simulink model "teseo"  (R2018a)
settings: Solver=FixedStepDiscrete  StartTime=0.0  StopTime=inf  FixedStep=0.1  RelTol=1e-3
model workspace (MAT data in the model file):
  SL_ROS_VariableLengthArrays_MaxSizes.CommonInfo.ArrayTruncateAction = 'EmitWarning'
  SL_ROS_VariableLengthArrays_MaxSizes.MsgTypeMap = containers.Map
  SL_ROS_VariableLengthArrays_MaxSizes.MsgTypeMap.serialization.keys = {'sensor_msgs/LaserScan'}
  SL_ROS_VariableLengthArrays_MaxSizes.MsgTypeMap.serialization.values{1}(1).PropertyName = 'Intensities'
  SL_ROS_VariableLengthArrays_MaxSizes.MsgTypeMap.serialization.values{1}(1).DataType = 'single'
  SL_ROS_VariableLengthArrays_MaxSizes.MsgTypeMap.serialization.values{1}(1).MaxLength = 360
  SL_ROS_VariableLengthArrays_MaxSizes.MsgTypeMap.serialization.values{1}(2).PropertyName = 'Ranges'
  SL_ROS_VariableLengthArrays_MaxSizes.MsgTypeMap.serialization.values{1}(2).DataType = 'single'
  SL_ROS_VariableLengthArrays_MaxSizes.MsgTypeMap.serialization.values{1}(2).MaxLength = 360
  SL_ROS_VariableLengthArrays_MaxSizes.MsgTypeMap.serialization.uniformity = 0
  SL_ROS_VariableLengthArrays_MaxSizes.MsgTypeMap.serialization.keyType = 'char'
  SL_ROS_VariableLengthArrays_MaxSizes.MsgTypeMap.serialization.valueType = 'any'
undefined symbols (not defined in the file or in its folder): Angular, anti_gain, Linear, max_vel
libraries: simulink x9, robotlib x5
settings Model: EnablePacing=on  PacingRate=10  Creator=Daniele  LastModifiedBy=gabriele
settings RTWCC: Description=Generic Real-Time Target  RTWCompilerOptimization=on
settings CodeAppCC: MaxIdLength=95  StateflowObjectComments=on

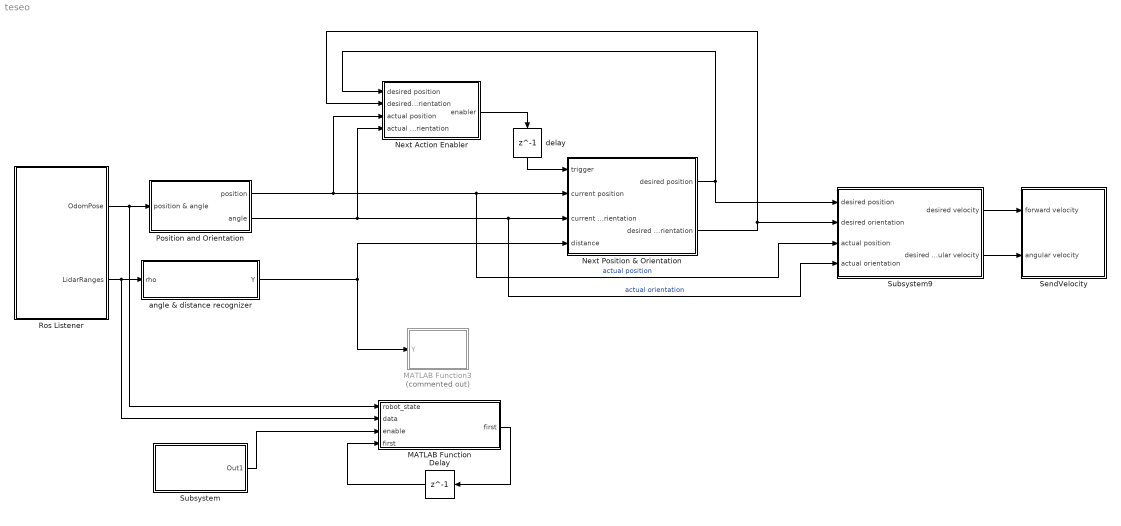
== system teseo ==
  Delay : Delay  DelayLength=1  InitialCondition=true
  MATLAB Function : MATLAB Function  TreatAsAtomicUnit=on
  MATLAB Function3 : MATLAB Function  Commented=on  TreatAsAtomicUnit=on
  Next Action Enabler : Subsystem
  Next Position & Orientation : Subsystem  mask{separation=0.5, offset=0, angle=2/9}
      mask prompts: separation "Distance between walls"; offset "Offset with respect to axes"; angle "Width of lateral angle: pi *"
  Position and Orientation : Subsystem
      mask Display:
      | disp('Pos/Angle\nSplitter')
      | port_label('input', 1, '[x y \theta]', 'interpreter', 'tex');
      | port_label('output', 1, '[x y]', 'interpreter', 'tex');
      | port_label('output', 2, '\theta', 'interpreter', 'tex');
  Ros Listener : Subsystem
  SendVelocity : Subsystem
  Subsystem : Subsystem
      mask Display: fprintf('Iteration Counter')
  Subsystem9 : Subsystem
  angle & distance recognizer : MATLAB Function  TreatAsAtomicUnit=on
  delay : Delay  DelayLength=1  InitialCondition=1
  wires:
  Ros Listener/1(OdomPose) -> MATLAB Function/1(robot_state), Position and Orientation/1(position & angle)
  Position and Orientation/1(position) -> Subsystem9/3(actual position), Next Position & Orientation/2(current position), Next Action Enabler/3(actual position)  "actual position"
  Position and Orientation/2(angle) -> Subsystem9/4(actual orientation), Next Position & Orientation/3(current orientation), Next Action Enabler/4(actual orientation)  "actual orientation"
  Ros Listener/2(LidarRanges) -> MATLAB Function/2(data), angle & distance recognizer/1(rho)
  angle & distance recognizer/1(Y) -> MATLAB Function3/1(Y), Next Position & Orientation/4(distance)
  delay/1 -> Next Position & Orientation/1(trigger)
  Next Action Enabler/1(enabler) -> delay/1
  Next Position & Orientation/1(desired position) -> Subsystem9/1(desired position), Next Action Enabler/1(desired position)
  Next Position & Orientation/2(desired orientation) -> Next Action Enabler/2(desired orientation), Subsystem9/2(desired orientation)
  Subsystem9/2(desired angular velocity) -> SendVelocity/2(angular velocity)
  Subsystem9/1(desired velocity) -> SendVelocity/1(forward velocity)
  Delay/1 -> MATLAB Function/4("first ")
  MATLAB Function/1(first) -> Delay/1
  Subsystem/1(Out1) -> MATLAB Function/3(enable)

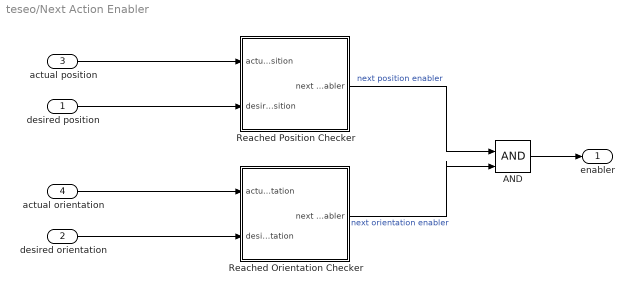
== system teseo/Next Action Enabler ==
  desired position : Inport
  desired orientation : Inport  Port=2
  actual position : Inport  Port=3
  actual orientation : Inport  Port=4
  AND : Logic  IconShape=distinctive  AllPortsSameDT=off  OutDataTypeStr=boolean
  Reached Orientation Checker : Subsystem  mask{stop_threshold=0.05, time_threshold=150}
      mask prompts: stop_threshold "Stop Threshold"; time_threshold "Time Threshold"
  Reached Position Checker : Subsystem  mask{stop_threshold=0.05, time_threshold=150}
      mask prompts: stop_threshold "Stop Treshold"; time_threshold "Time Treshold"
  enabler : Outport
  wires:
  actual orientation/1 -> Reached Orientation Checker/1(actual orientation)
  Reached Orientation Checker/1(next orientation enabler) -> AND/2  "next orientation enabler"
  Reached Position Checker/1(next position enabler) -> AND/1  "next position enabler"
  desired position/1 -> Reached Position Checker/2(desired position)
  desired orientation/1 -> Reached Orientation Checker/2(desired orientation)
  AND/1 -> enabler/1
  actual position/1 -> Reached Position Checker/1(actual position)

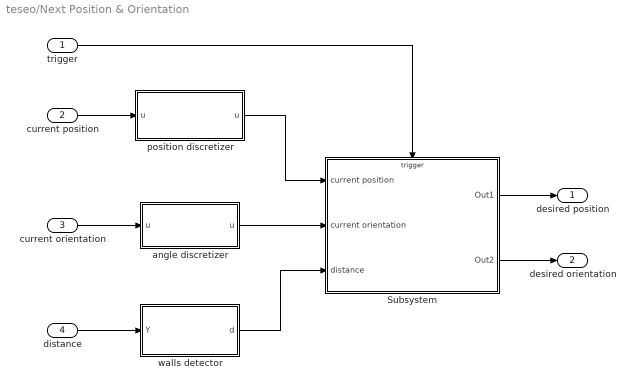
== system teseo/Next Position & Orientation ==
  trigger : Inport
  current position : Inport  Port=2
  current orientation : Inport  Port=3
  distance : Inport  Port=4
  Subsystem : Subsystem
  angle discretizer : MATLAB Function  TreatAsAtomicUnit=on
  position discretizer : MATLAB Function  TreatAsAtomicUnit=on  mask{width=separation, offset=offset}
      mask prompts: width "Distance between walls"; offset "Offset with respect to axes"
  walls detector : MATLAB Function  TreatAsAtomicUnit=on  mask{w=angle}
      mask prompts: w "Width of lateral angle"
  desired position : Outport
  desired orientation : Outport  Port=2
  wires:
  distance/1 -> walls detector/1(Y)
  current orientation/1 -> angle discretizer/1("u ")
  current position/1 -> position discretizer/1("u ")
  position discretizer/1(u) -> Subsystem/1(current position)
  angle discretizer/1(u) -> Subsystem/2(current orientation)
  walls detector/1(d) -> Subsystem/3(distance)
  Subsystem/1(Out1) -> desired position/1
  Subsystem/2(Out2) -> desired orientation/1
  trigger/1 -> Subsystem/Trigger

== system teseo/Position and Orientation ==
  position & angle : Inport
  Demux : Demux  Outputs=3
  Mux : Mux  Inputs=2
  position : Outport
  angle : Outport  Port=2
  wires:
  Demux/2 -> Mux/2
  position & angle/1 -> Demux/1
  Demux/1 -> Mux/1
  Mux/1 -> position/1
  Demux/3 -> angle/1

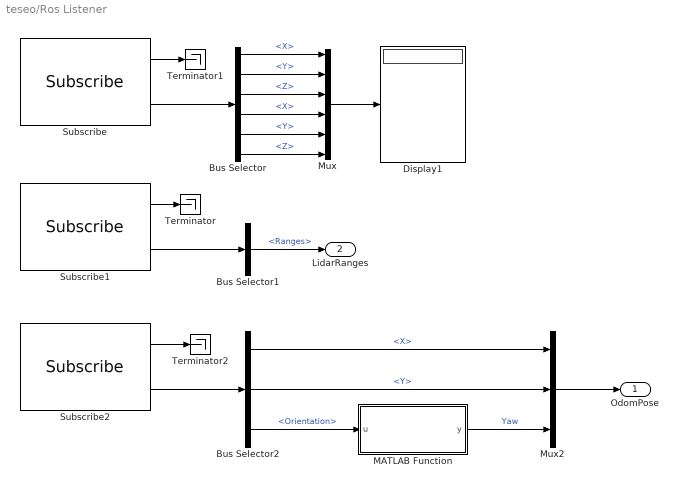
== system teseo/Ros Listener ==
  Bus Selector : BusSelector  OutputSignals=Linear.X,Linear.Y,Linear.Z,Angular.X,Angular.Y,Angular.Z
  Bus Selector1 : BusSelector  OutputSignals=Ranges
  Bus Selector2 : BusSelector  OutputSignals=Pose.Pose.Position.X,Pose.Pose.Position.Y,Pose.Pose.Orientation
  Display1 : Display
  MATLAB Function : MATLAB Function  TreatAsAtomicUnit=on
  Mux : Mux  Inputs=6
  Mux2 : Mux  Inputs=3
  Subscribe : robotlib/Subscribe  SourceLibraryInfo=This block requires Robotics System Toolbox  topicSource=Select from ROS network  topic=/mobile_base/commands/velocity  messageType=geometry_msgs/Twist  sampleTime=-1  messageQueueLength=1
      settings: SourceProductBaseCode=RO
  Subscribe1 : robotlib/Subscribe  SourceLibraryInfo=This block requires Robotics System Toolbox  topicSource=Select from ROS network  topic=/scan  messageType=sensor_msgs/LaserScan  sampleTime=-1  messageQueueLength=1
      settings: SourceProductBaseCode=RO
  Subscribe2 : robotlib/Subscribe  SourceLibraryInfo=This block requires Robotics System Toolbox  topicSource=Select from ROS network  topic=/odom  messageType=nav_msgs/Odometry  sampleTime=-1  messageQueueLength=1
      settings: SourceProductBaseCode=RO
  Terminator : Terminator
  Terminator1 : Terminator
  Terminator2 : Terminator
  OdomPose : Outport
  LidarRanges : Outport  Port=2
  wires:
  Bus Selector1/1 -> LidarRanges/1  "<Ranges>"
  Subscribe1/2 -> Bus Selector1/1
  Subscribe2/2 -> Bus Selector2/1
  Bus Selector2/1 -> Mux2/1  "<X>"
  Bus Selector2/2 -> Mux2/2  "<Y>"
  Mux2/1 -> OdomPose/1
  Bus Selector/5 -> Mux/5  "<Y>"
  Bus Selector/2 -> Mux/2  "<Y>"
  Bus Selector/1 -> Mux/1  "<X>"
  Bus Selector/6 -> Mux/6  "<Z>"
  Bus Selector/4 -> Mux/4  "<X>"
  Bus Selector/3 -> Mux/3  "<Z>"
  Mux/1 -> Display1/1
  Subscribe/2 -> Bus Selector/1
  Bus Selector2/3 -> MATLAB Function/1(u)  "<Orientation>"
  MATLAB Function/1(y) -> Mux2/3  "Yaw"
  Subscribe1/1 -> Terminator/1
  Subscribe/1 -> Terminator1/1
  Subscribe2/1 -> Terminator2/1

== system teseo/SendVelocity ==
  forward velocity : Inport
  angular velocity : Inport  Port=2
  Blank Message1 : robotlib/Blank Message  SourceLibraryInfo=This block requires Robotics System Toolbox  messageType=geometry_msgs/Twist  SampleTime=-1
      settings: SourceProductBaseCode=RO
  Bus Assignment1 : BusAssignment  AssignedSignals=Linear.X,Angular.Z
  Publish1 : robotlib/Publish  SourceLibraryInfo=This block requires Robotics System Toolbox  topicSource=Select from ROS network  topic=/cmd_vel  messageType=geometry_msgs/Twist  messageQueueLength=5
      settings: SourceProductBaseCode=RO
  wires:
  Blank Message1/1 -> Bus Assignment1/1
  forward velocity/1 -> Bus Assignment1/2
  angular velocity/1 -> Bus Assignment1/3
  Bus Assignment1/1 -> Publish1/1

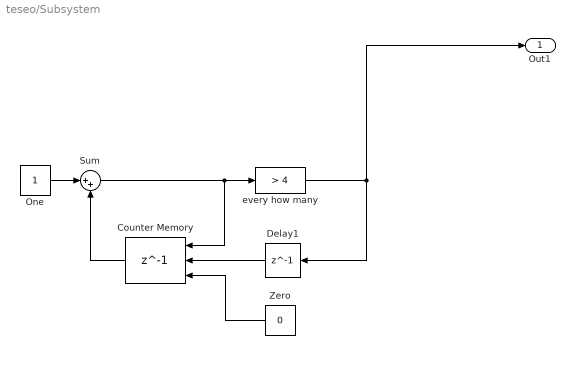
== system teseo/Subsystem ==
  Counter Memory : Delay  DelayLength=1  InitialConditionSource=Input port  ExternalReset=Rising
      settings: InputPortMap=u0,r5,p4
  Delay1 : Delay  DelayLength=1  InitialCondition=false
  One : Constant
  Sum : Sum  Inputs=|++
  Zero : Constant  Value=0
  every how many : simulink/Logic and Bit Operations/Compare To Constant  relop=>  const=4  OutDataTypeStr=boolean
  Out1 : Outport
  wires:
  Zero/1 -> Counter Memory/3
  Sum/1 -> every how many/1, Counter Memory/1
  Delay1/1 -> Counter Memory/2
  Counter Memory/1 -> Sum/2
  every how many/1 -> Out1/1, Delay1/1
  One/1 -> Sum/1

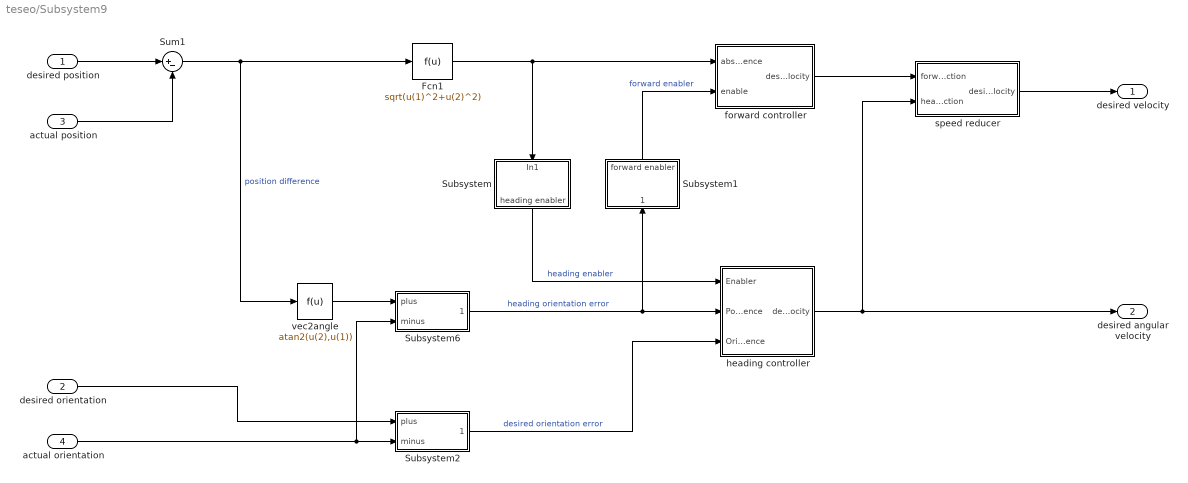
== system teseo/Subsystem9 ==
  desired position : Inport
  desired orientation : Inport  Port=2
  actual position : Inport  Port=3
  actual orientation : Inport  Port=4
  Fcn1 : Fcn  Expr=sqrt(u(1)^2+u(2)^2)
      mask Display: disp('norm')
  Subsystem : Subsystem  mask{heading_en_threshold=0.05}
      mask prompts: heading_en_threshold "Heading Enabler Threshold: |u| >"
      mask Display: fprintf("Heading\nEnabler")
  Subsystem1 : Subsystem  mask{forward_en_threshold=0.2}
      mask prompts: forward_en_threshold "Forward Motion Enabler Threshold: |u| <"
      mask Display: fprintf("Forward\nEnabler")
  Subsystem2 : Subsystem
      mask Display:
      | disp('anglediff');
      | port_label('input', 1, '+');
      | port_label('input', 2, '-');
  Subsystem6 : Subsystem
      mask Display:
      | disp('anglediff');
      | port_label('input', 1, '+');
      | port_label('input', 2, '-');
  Sum1 : Sum  Inputs=|+-
  forward controller : Subsystem  mask{gain=2, int_gain=0, der_gain=0.5}
      mask prompts: gain "Proportional Gain"; int_gain "Integral Gain"; der_gain "Derivative Gain"
      mask Display: disp('Forward Motion\nController')
  heading controller : Subsystem  mask{gain=2, int_gain=0, der_gain=1}
      mask prompts: gain "Proportional Gain"; int_gain "Integral Gain"; der_gain "Derivative Gain"
      mask Display: disp('Yaw Controller')
  speed reducer : Subsystem  mask{speed_red_threshold=0.5, low_speed=0.5, high_speed=0.75}
      mask prompts: speed_red_threshold "Speed Reducer Threshold: |heading action| >"; low_speed "Low Speed Multiplier"; high_speed "High Speed Multiplier"
      mask Display: fprintf("Speed Reducer")
  vec2angle : Fcn  Expr=atan2(u(2),u(1))
      mask Display: disp('angle')
  desired velocity : Outport
  desired angular velocity : Outport  Port=2
  wires:
  vec2angle/1 -> Subsystem6/1("plus ")
  heading controller/1(desired angular velocity) -> speed reducer/2(heading action), desired angular velocity/1
  actual orientation/1 -> Subsystem2/2(minus), Subsystem6/2(minus)
  desired orientation/1 -> Subsystem2/1("plus ")
  desired position/1 -> Sum1/1
  Sum1/1 -> vec2angle/1, Fcn1/1  "position difference"
  Subsystem2/1(difference) -> heading controller/3(Orientation Angular Difference)  "desired orientation error"
  actual position/1 -> Sum1/2
  Fcn1/1 -> Subsystem/1(In1), forward controller/1(absolute position difference)
  Subsystem6/1(difference) -> heading controller/2(Position Angular Difference), Subsystem1/1(heading orientation error)  "heading orientation error"
  forward controller/1(desired velocity) -> speed reducer/1(forward action)
  speed reducer/1(desired velocity) -> desired velocity/1
  Subsystem/1(heading enabler) -> heading controller/1(Enabler)  "heading enabler"
  Subsystem1/1(forward enabler) -> forward controller/2(enable)  "forward enabler"

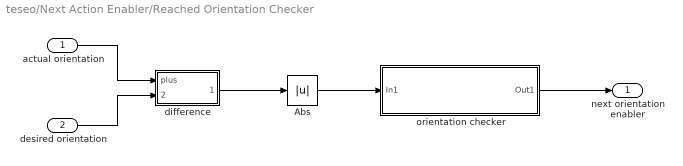
== system teseo/Next Action Enabler/Reached Orientation Checker ==
  actual orientation : Inport
  desired orientation : Inport  Port=2
  Abs : Abs
  difference : Subsystem
      mask Display: disp('anglediff')
  orientation checker : Subsystem  mask{stop_treshold=stop_threshold, time_threshold=time_threshold}
      mask prompts: stop_treshold "Stop Threshold"; time_threshold "Time Threshold"
      mask Display: fprintf("Reached Destination Checker");
  next orientation enabler : Outport
  wires:
  difference/1(difference) -> Abs/1
  Abs/1 -> orientation checker/1(In1)
  orientation checker/1(Out1) -> next orientation enabler/1
  actual orientation/1 -> difference/1("plus ")
  desired orientation/1 -> difference/2(minus)

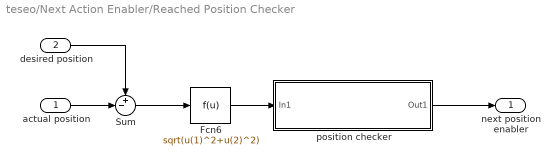
== system teseo/Next Action Enabler/Reached Position Checker ==
  actual position : Inport
  desired position : Inport  Port=2
  Fcn6 : Fcn  Expr=sqrt(u(1)^2+u(2)^2)
      mask Display: disp('norm')
  Sum : Sum  Inputs=+-|
  position checker : Subsystem  mask{stop_treshold=stop_threshold, time_threshold=time_threshold}
      mask prompts: stop_treshold "Stop Threshold"; time_threshold "Time Threshold"
      mask Display: fprintf("Reached Destination Checker");
  next position enabler : Outport
  wires:
  Fcn6/1 -> position checker/1(In1)
  Sum/1 -> Fcn6/1
  actual position/1 -> Sum/2
  desired position/1 -> Sum/1
  position checker/1(Out1) -> next position enabler/1

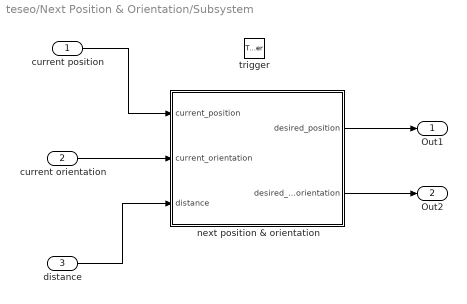
== system teseo/Next Position & Orientation/Subsystem ==
  current position : Inport
  current orientation : Inport  Port=2
  distance : Inport  Port=3
  trigger : TriggerPort  VariantControl=Variant  InitialTriggerSignalState=zero  PortDimensions=1
  next position & orientation : MATLAB Function  TreatAsAtomicUnit=on
  Out1 : Outport
  Out2 : Outport  Port=2
  wires:
  current orientation/1 -> next position & orientation/2(current_orientation)
  distance/1 -> next position & orientation/3(distance)
  next position & orientation/2(desired_orientation) -> Out2/1
  next position & orientation/1(desired_position) -> Out1/1
  current position/1 -> next position & orientation/1(current_position)

== system teseo/Subsystem9/Subsystem ==
  In1 : Inport
  Abs : Abs
  Compare To Constant : simulink/Logic and Bit Operations/Compare To Constant  relop=>  const=heading_en_threshold  OutDataTypeStr=boolean
  heading enabler : Outport
  wires:
  Compare To Constant/1 -> heading enabler/1
  In1/1 -> Abs/1
  Abs/1 -> Compare To Constant/1

== system teseo/Subsystem9/Subsystem1 ==
  heading orientation error : Inport
  Abs : Abs
  Compare To Constant : simulink/Logic and Bit Operations/Compare To Constant  relop=<  const=forward_en_threshold  OutDataTypeStr=boolean
  forward enabler : Outport
  wires:
  heading orientation error/1 -> Abs/1
  Compare To Constant/1 -> forward enabler/1
  Abs/1 -> Compare To Constant/1

== system teseo/Subsystem9/Subsystem2 ==
  "plus " : Inport
  minus : Inport  Port=2
  MATLAB Function : MATLAB Function  TreatAsAtomicUnit=on
  Mux : Mux  Inputs=2
  difference : Outport
  wires:
  MATLAB Function/1(y) -> difference/1
  Mux/1 -> MATLAB Function/1(u)
  "plus "/1 -> Mux/2
  minus/1 -> Mux/1

== system teseo/Subsystem9/Subsystem6 ==
  "plus " : Inport
  minus : Inport  Port=2
  MATLAB Function : MATLAB Function  TreatAsAtomicUnit=on
  Mux : Mux  Inputs=2
  difference : Outport
  wires:
  MATLAB Function/1(y) -> difference/1
  Mux/1 -> MATLAB Function/1(u)
  "plus "/1 -> Mux/2
  minus/1 -> Mux/1

== system teseo/Subsystem9/forward controller ==
  absolute position difference : Inport
  enable : Inport  Port=2
  PID Controller : simulink/Continuous/PID Controller  Controller=PID  TimeDomain=Discrete-time  SampleTime=-1  IntegratorMethod=Forward Euler  FilterMethod=Trapezoidal  Form=Parallel  UseFilter=on  ControllerParametersSource=internal  P=gain  I=int_gain  D=der_gain  N=100  InitialConditionSource=internal  InitialConditionForIntegrator=0  InitialConditionForFilter=0  ExternalReset=none  LimitOutput=off  UpperSaturationLimit=max_vel  LowerSaturationLimit=-max_vel  LinearizeAsGain=on  AntiWindupMode=back-calculation  Kb=anti_gain  TrackingMode=off  Kt=1  PParamMin=[]  PParamMax=[]  IParamMin=[]  IParamMax=[]  DParamMin=[]  DParamMax=[]  NParamMin=[]  NParamMax=[]  KbParamMin=[]  KbParamMax=[]  KtParamMin=[]  KtParamMax=[]  POutMin=[]  POutMax=[]  IOutMin=[]  IOutMax=[]  DOutMin=[]  DOutMax=[]  NOutMin=[]  NOutMax=[]  KbOutMin=[]  KbOutMax=[]  KtOutMin=[]  KtOutMax=[]  IntegratorOutMin=[]  IntegratorOutMax=[]  FilterOutMin=[]  FilterOutMax=[]  SumOutMin=[]  SumOutMax=[]  SumI1OutMin=[]  SumI1OutMax=[]  SumI2OutMin=[]  SumI2OutMax=[]  SumI3OutMin=[]  SumI3OutMax=[]  SumDOutMin=[]  SumDOutMax=[]  SaturationOutMin=[]  SaturationOutMax=[]  IntegratorContinuousStateAttributes=''  IntegratorStateMustResolveToSignalObject=off  IntegratorRTWStateStorageClass=Auto  FilterContinuousStateAttributes=''  FilterStateMustResolveToSignalObject=off  FilterRTWStateStorageClass=Auto  DifferentiatorICPrevScaledInput=0  DifferentiatorOutMin=[]  DifferentiatorOutMax=[]  FilterDiffOutCoefMin=[]  FilterDiffOutCoefMax=[]  SumDenOutMin=[]  SumDenOutMax=[]  SumNumOutMin=[]  SumNumOutMax=[]  ReciprocalOutMin=[]  ReciprocalOutMax=[]  DivideOutMin=[]  DivideOutMax=[]  TunerSelectOption=Frequency Response Based
  Switch2 : Switch
  zero : Constant  Value=0
  desired velocity : Outport
  wires:
  zero/1 -> Switch2/3
  Switch2/1 -> PID Controller/1
  enable/1 -> Switch2/2
  absolute position difference/1 -> Switch2/1
  PID Controller/1 -> desired velocity/1

== system teseo/Subsystem9/heading controller ==
  Enabler : Inport
  Position Angular Difference : Inport  Port=2
  Orientation Angular Difference : Inport  Port=3
  PID Controller : simulink/Continuous/PID Controller  Controller=PID  TimeDomain=Discrete-time  SampleTime=-1  IntegratorMethod=Trapezoidal  FilterMethod=Trapezoidal  Form=Parallel  UseFilter=on  ControllerParametersSource=internal  P=gain  I=int_gain  D=der_gain  N=100  InitialConditionSource=internal  InitialConditionForIntegrator=0  InitialConditionForFilter=0  ExternalReset=none  LimitOutput=off  UpperSaturationLimit=inf  LowerSaturationLimit=-inf  LinearizeAsGain=on  AntiWindupMode=none  Kb=1  TrackingMode=off  Kt=1  PParamMin=[]  PParamMax=[]  IParamMin=[]  IParamMax=[]  DParamMin=[]  DParamMax=[]  NParamMin=[]  NParamMax=[]  KbParamMin=[]  KbParamMax=[]  KtParamMin=[]  KtParamMax=[]  POutMin=[]  POutMax=[]  IOutMin=[]  IOutMax=[]  DOutMin=[]  DOutMax=[]  NOutMin=[]  NOutMax=[]  KbOutMin=[]  KbOutMax=[]  KtOutMin=[]  KtOutMax=[]  IntegratorOutMin=[]  IntegratorOutMax=[]  FilterOutMin=[]  FilterOutMax=[]  SumOutMin=[]  SumOutMax=[]  SumI1OutMin=[]  SumI1OutMax=[]  SumI2OutMin=[]  SumI2OutMax=[]  SumI3OutMin=[]  SumI3OutMax=[]  SumDOutMin=[]  SumDOutMax=[]  SaturationOutMin=[]  SaturationOutMax=[]  IntegratorContinuousStateAttributes=''  IntegratorStateMustResolveToSignalObject=off  IntegratorRTWStateStorageClass=Auto  FilterContinuousStateAttributes=''  FilterStateMustResolveToSignalObject=off  FilterRTWStateStorageClass=Auto  DifferentiatorICPrevScaledInput=0  DifferentiatorOutMin=[]  DifferentiatorOutMax=[]  FilterDiffOutCoefMin=[]  FilterDiffOutCoefMax=[]  SumDenOutMin=[]  SumDenOutMax=[]  SumNumOutMin=[]  SumNumOutMax=[]  ReciprocalOutMin=[]  ReciprocalOutMax=[]  DivideOutMin=[]  DivideOutMax=[]  TunerSelectOption=Frequency Response Based
  Switch : Switch
  desired angular velocity : Outport
  wires:
  Position Angular Difference/1 -> Switch/1
  PID Controller/1 -> desired angular velocity/1
  Switch/1 -> PID Controller/1
  Orientation Angular Difference/1 -> Switch/3
  Enabler/1 -> Switch/2

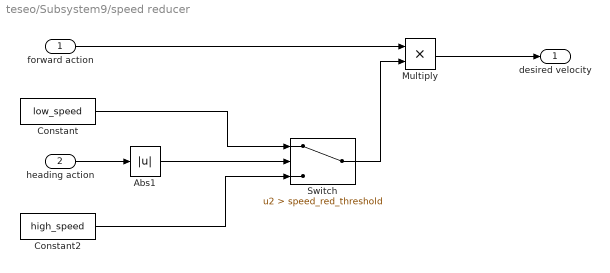
== system teseo/Subsystem9/speed reducer ==
  forward action : Inport
  heading action : Inport  Port=2
  Abs1 : Abs
  Constant : Constant  Value=low_speed
  Constant2 : Constant  Value=high_speed
  Multiply : Product
  Switch : Switch  Criteria=u2 > Threshold  Threshold=speed_red_threshold
  desired velocity : Outport
  wires:
  forward action/1 -> Multiply/1
  Switch/1 -> Multiply/2
  Constant2/1 -> Switch/3
  Multiply/1 -> desired velocity/1
  heading action/1 -> Abs1/1
  Abs1/1 -> Switch/2
  Constant/1 -> Switch/1

== system teseo/Next Action Enabler/Reached Orientation Checker/difference ==
  "plus " : Inport
  minus : Inport  Port=2
  MATLAB Function : MATLAB Function  TreatAsAtomicUnit=on
  Mux : Mux  Inputs=2
  difference : Outport
  wires:
  MATLAB Function/1(y) -> difference/1
  Mux/1 -> MATLAB Function/1(u)
  "plus "/1 -> Mux/2
  minus/1 -> Mux/1

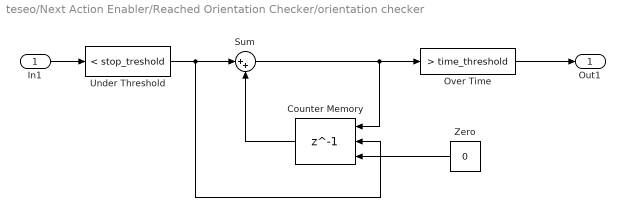
== system teseo/Next Action Enabler/Reached Orientation Checker/orientation checker ==
  In1 : Inport
  Counter Memory : Delay  DelayLength=1  InitialConditionSource=Input port  ExternalReset=Falling
      settings: InputPortMap=u0,r5,p4
  Over Time : simulink/Logic and Bit Operations/Compare To Constant  relop=>  const=time_threshold  OutDataTypeStr=boolean
  Sum : Sum  Inputs=|++
  Under Threshold : simulink/Logic and Bit Operations/Compare To Constant  relop=<  const=stop_treshold  OutDataTypeStr=uint8
  Zero : Constant  Value=0
  Out1 : Outport
  wires:
  Zero/1 -> Counter Memory/3
  Under Threshold/1 -> Sum/1, Counter Memory/2
  In1/1 -> Under Threshold/1
  Counter Memory/1 -> Sum/2
  Sum/1 -> Over Time/1, Counter Memory/1
  Over Time/1 -> Out1/1

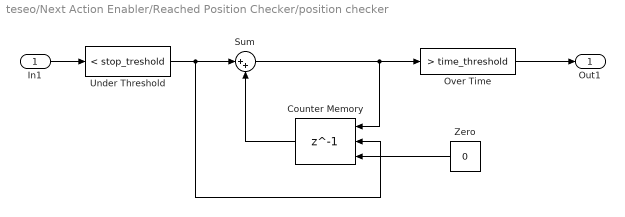
== system teseo/Next Action Enabler/Reached Position Checker/position checker ==
  In1 : Inport
  Counter Memory : Delay  DelayLength=1  InitialConditionSource=Input port  ExternalReset=Falling
      settings: InputPortMap=u0,r5,p4
  Over Time : simulink/Logic and Bit Operations/Compare To Constant  relop=>  const=time_threshold  OutDataTypeStr=boolean
  Sum : Sum  Inputs=|++
  Under Threshold : simulink/Logic and Bit Operations/Compare To Constant  relop=<  const=stop_treshold  OutDataTypeStr=uint8
  Zero : Constant  Value=0
  Out1 : Outport
  wires:
  Zero/1 -> Counter Memory/3
  Under Threshold/1 -> Sum/1, Counter Memory/2
  In1/1 -> Under Threshold/1
  Counter Memory/1 -> Sum/2
  Sum/1 -> Over Time/1, Counter Memory/1
  Over Time/1 -> Out1/1

== matlab function teseo/Subsystem9/Subsystem2/MATLAB Function ==
  data: u input; y output
function y = fcn(u)

y = angdiff(u);

== matlab function teseo/MATLAB Function ==
  data: robot_state input; data input; enable input boolean; first input boolean; first output
function first  = print2file(robot_state, data, enable,first)
%#codegen

%coder.extrinsic('fopen');

if ~enable
    return;
end

filename = 'log.txt';

if first
    first = false;
    file = fopen(filename, 'w');
else
    file = fopen(filename, 'a');
end

fprintf(file, '%f\t%f\t%f', robot_state(1), robot_state(2), robot_state(3));

for j = 1:length(data)
    fprintf(file, '\t%f', data(j));
end

fprintf(file, '\r\n');
fclose(file);

end

== matlab function teseo/Next Position & Orientation/Subsystem/next position & orientation ==
  data: current_position input; desired_position output; current_orientation input; distance input; desired_orientation output; separation parameter
function [desired_position, desired_orientation] = next_position(current_position, current_orientation, distance, separation)

t = within_PI_PI(current_orientation);

W = distance(1);
N = distance(2);
E = distance(3);
S = distance(4);

R = [...
    cos(t) -sin(t)  0;
    sin(t)  cos(t)  0;
    0       0       1
    ];

if W > separation
    d = [0; 1; 0];
    t = t + pi/2;
elseif N > separation
    d = [1; 0; 0];
    % t = t;
elseif E > separation
    d = [0; -1; 0];
    t = t - pi/2;
elseif S > separation
    d = [-1; 0; 0];
    t = t + pi;
else
    % STOP - should never happen
    d = [0; 0; 0];
    
    % t = current_orientation;
end

d = d * separation;

d = R * d;
desired_position = current_position + d(1:2);

desired_orientation = within_PI_PI(t);

% desired_position = current_position;
% desired_orientation = current_orientation;

end

function t = within_PI_PI(t)

if t > pi
    t = t - 2*pi;
elseif t < -pi
    t = t + 2*pi;
end

end

== matlab function teseo/Ros Listener/MATLAB Function ==
  data: u input; y output
function y = Orientation2Yaw(u)

x = quat2eul([u.W u.X u.Y u.Z]);
y = x(1);

== matlab function teseo/angle & distance recognizer ==
  data: Y output; rho input
function Y = angle_distance_recognizer(rho)

N = length(rho);
alpha = (0:N-1);
alpha = alpha * pi * 2 / N;

Y = [rho'; alpha];

== matlab function teseo/Next Position & Orientation/walls detector ==
  data: Y input; d output; w parameter
function d = distance_WNES(Y, w)

W_less = pi * (1/2  - w/2);
W_more = pi * (1/2  + w/2);
N_less = pi * (2    - w/2);
N_more = pi * (0    + w/2);
E_less = pi * (3/2  - w/2);
E_more = pi * (3/2  + w/2);
S_less = pi * (1    - w/2);
S_more = pi * (1    + w/2);

W_idx = and(Y(2, :) > W_less, Y(2, :) < W_more);
N_idx = or( Y(2, :) > N_less, Y(2, :) < N_more);
E_idx = and(Y(2, :) > E_less, Y(2, :) < E_more);
S_idx = and(Y(2, :) > S_less, Y(2, :) < S_more);

W = Y(1, W_idx);
N = Y(1, N_idx);
E = Y(1, E_idx);
S = Y(1, S_idx);

d = [...
    median(W)
    median(N)
    median(E)
    median(S)
    ];

end

== matlab function teseo/MATLAB Function3 ==
  data: Y input
function fcn(Y)

x = Y(1, :) .* cos(Y(2, :));
y = Y(1, :) .* sin(Y(2, :));

plot(x,y,"+r");

== matlab function teseo/Next Action Enabler/Reached Orientation Checker/difference/MATLAB Function ==
  data: u input; y output
function y = fcn(u)

y = angdiff(u);

== matlab function teseo/Next Position & Orientation/position discretizer ==
  data: u input; u output; offset parameter; width parameter
function u = position_discretizer(u, offset, width)

u = round((u - offset) / width) * width + offset;

== matlab function teseo/Next Position & Orientation/angle discretizer ==
  data: u input; u output
function u = angle_discretizer(u)

PI_2 = pi/2;

u = round(u / PI_2) * PI_2;

end

== matlab function teseo/Subsystem9/Subsystem6/MATLAB Function ==
  data: u input; y output
function y = fcn(u)

y = angdiff(u);
